simulink library "HEV_Battery_Lib"  (R2024b)
settings: Solver=ode45  StartTime=0.0  StopTime=10.0  RelTol=1e-3  EnableMultiTasking=on
undefined symbols (not defined in the file or in its folder): HEV_Param, Hydride, Kt_Temps, Metal, Nickel
libraries: fl_lib x58, nesl_utility x35, LeadAcidBattery_lib x8, $bdroot x5, Rcecm_lib x4, batteryecm_lib x3, Capacitors_lib x1, spsBatteryLib x1, simulink_extras x1, spsGroundLib x1, spsControlledCurrentSourceLib x1, spsVoltageMeasurementLib x1
(part 2 of 2)

== system HEV_Battery_Lib/Cells/Battery cell2/Thermal Model ==
  Battery thermal mass : fl_lib/Thermal/Thermal Elements/Thermal Mass  mass_type=foundation.enum.constant_variable.constant  mass=1 kg  sp_heat=HEV_Param.Battery_Cell.Ctheta J/kg/K  mass_min=1e-6 kg  num_ports=foundation.enum.numPorts2.one  m_specify=off  m_priority=High  m=1 kg  m_nominal_specify=off  m_nominal_value=1  m_nominal_unit=kg  T_specify=on  T_priority=High  T=HEV_Param.Battery_Cell.theta_init+273 K  T_nominal_specify=off  T_nominal_value=1  T_nominal_unit=K  Q_specify=off  Q_priority=High  Q=0 J/s  Q_nominal_specify=off  Q_nominal_value=1  Q_nominal_unit=J/s
  Ideal Temperature Sensor : fl_lib/Thermal/Thermal Sensors/Temperature Sensor  temperature_measure=foundation.enum.MeasurementReference.difference
  Ideal Heat Flow Source : fl_lib/Thermal/Thermal Sources/Controlled Heat Flow Rate Source
  Kt as a function of temperature : fl_lib/Physical Signals/Lookup Tables/PS Lookup Table (1D)  x=[HEV_Param.Battery_Cell.theta_f,HEV_Param.Battery_Cell. Kt_Temps]+273 K  f=[0 HEV_Param.Battery_Cell.Kt]  interp_method=simscape.enum.interpolation.linear  extrap_method=simscape.enum.extrapolation.linear
  Thermal Reference1 : fl_lib/Thermal/Thermal Elements/Thermal Reference
  Thermal Reference2 : fl_lib/Thermal/Thermal Elements/Thermal Reference
  Ps : PMIOPort  Tag=PMCPort  Side=Left
  H : PMIOPort  Tag=PMCPort  Port=2  Side=Left
  Kt : PMIOPort  Tag=PMCPort  Port=3  Side=Right
  T : PMIOPort  Tag=PMCPort  Port=4  Side=Right
  connections:
  Ideal Heat Flow Source/RConn1 -- Ps/RConn1
  Kt/RConn1 -- Kt as a function of temperature/RConn1
  Battery thermal mass/LConn1 -- Ideal Heat Flow Source/LConn1 -- Ideal Temperature Sensor/LConn1 -- H/RConn1
  Thermal Reference1/LConn1 -- Ideal Heat Flow Source/RConn2
  T/RConn1 -- Kt as a function of temperature/LConn1 -- Ideal Temperature Sensor/RConn2
  Ideal Temperature Sensor/RConn1 -- Thermal Reference2/LConn1

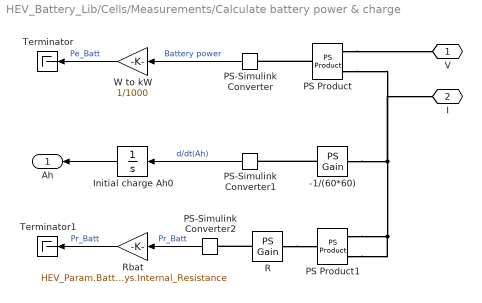
== system HEV_Battery_Lib/Cells/Measurements/Calculate battery power & charge ==
  -1/(60*60) : fl_lib/Physical Signals/Functions/PS Gain  gain=-1/(60*60)
  Initial charge Ah0 : Integrator  InitialCondition=HEV_Param.Battery_Sys.Maximum_Capacity
  PS Product : fl_lib/Physical Signals/Functions/PS Product
  PS Product1 : fl_lib/Physical Signals/Functions/PS Product
  PS-Simulink Converter : nesl_utility/PS-Simulink Converter  PhysicalDomain=network_engine_domain  SubClassName=ps_output  LeftPortType=input  RightPortType=output  PseudoPeriodic=off  Frequencies=[]  VectorFormat=1-D array  Unit=W  AffineConversion=off
  PS-Simulink Converter1 : nesl_utility/PS-Simulink Converter  PhysicalDomain=network_engine_domain  SubClassName=ps_output  LeftPortType=input  RightPortType=output  PseudoPeriodic=off  Frequencies=[]  VectorFormat=1-D array  Unit=A  AffineConversion=off
  PS-Simulink Converter2 : nesl_utility/PS-Simulink Converter  PhysicalDomain=network_engine_domain  SubClassName=ps_output  LeftPortType=input  RightPortType=output  PseudoPeriodic=off  Frequencies=[]  VectorFormat=1-D array  Unit=W  AffineConversion=off
  R : fl_lib/Physical Signals/Functions/PS Gain  gain=HEV_Param.Battery_Sys.Internal_Resistance Ohm
  Rbat : Gain  Gain=HEV_Param.Battery_Sys.Internal_Resistance
  Terminator : Terminator
  Terminator1 : Terminator
  W to kW : Gain  Gain=1/1000
  V : PMIOPort  Side=Left
  I : PMIOPort  Port=2  Side=Left
  Ah : Outport  VectorParamsAs1DForOutWhenUnconnected=off
  wires:
  Rbat/1 -> Terminator1/1  "Pr_Batt"
  Initial charge Ah0/1 -> Ah/1
  W to kW/1 -> Terminator/1  "Pe_Batt"
  PS-Simulink Converter1/1 -> Initial charge Ah0/1  "d/dt(Ah)"
  PS-Simulink Converter2/1 -> Rbat/1  "Pr_Batt"
  PS-Simulink Converter/1 -> W to kW/1  "Battery power"
  connections:
  -1/(60*60)/LConn1 -- PS Product/LConn2 -- I/RConn1 -- PS Product1/LConn2 -- PS Product1/LConn1
  PS Product/LConn1 -- V/RConn1
  R/LConn1 -- PS Product1/RConn1
  -1/(60*60)/RConn1 -- PS-Simulink Converter1/LConn1
  R/RConn1 -- PS-Simulink Converter2/LConn1
  PS Product/RConn1 -- PS-Simulink Converter/LConn1

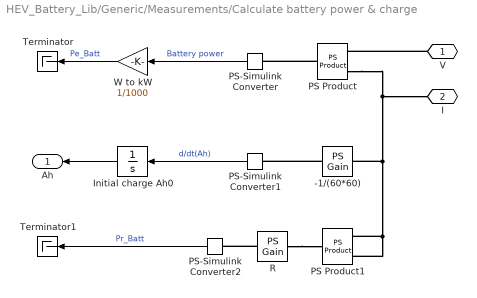
== system HEV_Battery_Lib/Generic/Measurements/Calculate battery power & charge ==
  -1/(60*60) : fl_lib/Physical Signals/Functions/PS Gain  gain=-1/(60*60)
  Initial charge Ah0 : Integrator  InitialCondition=HEV_Param.Battery_Sys.Maximum_Capacity
  PS Product : fl_lib/Physical Signals/Functions/PS Product
  PS Product1 : fl_lib/Physical Signals/Functions/PS Product
  PS-Simulink Converter : nesl_utility/PS-Simulink Converter  PhysicalDomain=network_engine_domain  SubClassName=ps_output  LeftPortType=input  RightPortType=output  PseudoPeriodic=off  Frequencies=[]  VectorFormat=1-D array  Unit=W  AffineConversion=off
  PS-Simulink Converter1 : nesl_utility/PS-Simulink Converter  PhysicalDomain=network_engine_domain  SubClassName=ps_output  LeftPortType=input  RightPortType=output  PseudoPeriodic=off  Frequencies=[]  VectorFormat=1-D array  Unit=A  AffineConversion=off
  PS-Simulink Converter2 : nesl_utility/PS-Simulink Converter  PhysicalDomain=network_engine_domain  SubClassName=ps_output  LeftPortType=input  RightPortType=output  PseudoPeriodic=off  Frequencies=[]  VectorFormat=1-D array  Unit=W  AffineConversion=off
  R : fl_lib/Physical Signals/Functions/PS Gain  gain=HEV_Param.Battery_Sys.Internal_Resistance Ohm
  Terminator : Terminator
  Terminator1 : Terminator
  W to kW : Gain  Gain=1/1000
  V : PMIOPort  Side=Left
  I : PMIOPort  Port=2  Side=Left
  Ah : Outport  VectorParamsAs1DForOutWhenUnconnected=off
  wires:
  PS-Simulink Converter/1 -> W to kW/1  "Battery power"
  W to kW/1 -> Terminator/1  "Pe_Batt"
  PS-Simulink Converter1/1 -> Initial charge Ah0/1  "d/dt(Ah)"
  Initial charge Ah0/1 -> Ah/1
  PS-Simulink Converter2/1 -> Terminator1/1  "Pr_Batt"
  connections:
  R/RConn1 -- PS-Simulink Converter2/LConn1
  PS Product/RConn1 -- PS-Simulink Converter/LConn1
  V/RConn1 -- PS Product/LConn1
  PS Product/LConn2 -- I/RConn1 -- -1/(60*60)/LConn1 -- PS Product1/LConn1 -- PS Product1/LConn2
  -1/(60*60)/RConn1 -- PS-Simulink Converter1/LConn1
  R/LConn1 -- PS Product1/RConn1

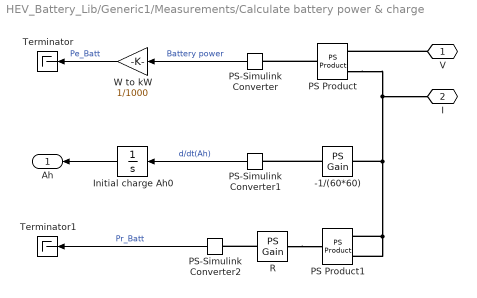
== system HEV_Battery_Lib/Generic1/Measurements/Calculate battery power & charge ==
  -1/(60*60) : fl_lib/Physical Signals/Functions/PS Gain  gain=-1/(60*60)
  Initial charge Ah0 : Integrator  InitialCondition=HEV_Param.Battery_Sys.Maximum_Capacity
  PS Product : fl_lib/Physical Signals/Functions/PS Product
  PS Product1 : fl_lib/Physical Signals/Functions/PS Product
  PS-Simulink Converter : nesl_utility/PS-Simulink Converter  PhysicalDomain=network_engine_domain  SubClassName=ps_output  LeftPortType=input  RightPortType=output  PseudoPeriodic=off  Frequencies=[]  VectorFormat=1-D array  Unit=W  AffineConversion=off
  PS-Simulink Converter1 : nesl_utility/PS-Simulink Converter  PhysicalDomain=network_engine_domain  SubClassName=ps_output  LeftPortType=input  RightPortType=output  PseudoPeriodic=off  Frequencies=[]  VectorFormat=1-D array  Unit=A  AffineConversion=off
  PS-Simulink Converter2 : nesl_utility/PS-Simulink Converter  PhysicalDomain=network_engine_domain  SubClassName=ps_output  LeftPortType=input  RightPortType=output  PseudoPeriodic=off  Frequencies=[]  VectorFormat=1-D array  Unit=W  AffineConversion=off
  R : fl_lib/Physical Signals/Functions/PS Gain  gain=HEV_Param.Battery_Sys.Internal_Resistance Ohm
  Terminator : Terminator
  Terminator1 : Terminator
  W to kW : Gain  Gain=1/1000
  V : PMIOPort  Side=Left
  I : PMIOPort  Port=2  Side=Left
  Ah : Outport  VectorParamsAs1DForOutWhenUnconnected=off
  wires:
  PS-Simulink Converter/1 -> W to kW/1  "Battery power"
  W to kW/1 -> Terminator/1  "Pe_Batt"
  PS-Simulink Converter1/1 -> Initial charge Ah0/1  "d/dt(Ah)"
  Initial charge Ah0/1 -> Ah/1
  PS-Simulink Converter2/1 -> Terminator1/1  "Pr_Batt"
  connections:
  R/RConn1 -- PS-Simulink Converter2/LConn1
  PS Product/RConn1 -- PS-Simulink Converter/LConn1
  V/RConn1 -- PS Product/LConn1
  PS Product/LConn2 -- I/RConn1 -- -1/(60*60)/LConn1 -- PS Product1/LConn1 -- PS Product1/LConn2
  -1/(60*60)/RConn1 -- PS-Simulink Converter1/LConn1
  R/LConn1 -- PS Product1/RConn1

== system HEV_Battery_Lib/Predefined/GF1/SOC Offset ==
  note: For control logic to work consistently
      | for all versions, SOC% must be scaled
  In1 : Inport
  Bus Creator : BusCreator  Inputs=4
  Bus Selector : BusSelector  OutputSignals=SOC (%)
  Bus Selector1 : BusSelector  OutputSignals=Current (A),Voltage (V)
  Gain : Gain  Gain=100/HEV_Param.Battery_Det.Initial_SOC
  Gain1 : Gain  Gain=-1/(60*60)
  Initial charge Ah0 : Integrator  InitialCondition=HEV_Param.Battery_Det.Rated_Capacity*HEV_Param.Battery_Det.Initial_SOC/100
  Transfer Fcn (with initial states) : simulink_extras/Additional Linear/Transfer Fcn (with initial states)  N=[1]  D="[0.01  1]"  X0=100/HEV_Param.Battery_Det.Initial_SOC
  Out1 : Outport  VectorParamsAs1DForOutWhenUnconnected=off
  wires:
  In1/1 -> Bus Selector/1, Bus Selector1/1
  Bus Selector/1 -> Gain/1  "<SOC (%)>"
  Bus Selector1/1 -> Bus Creator/2, Gain1/1  "<Current (A)>"
  Gain/1 -> Transfer Fcn (with initial states)/1  "SOC (%)"
  Bus Selector1/2 -> Bus Creator/3  "<Voltage (V)>"
  Bus Creator/1 -> Out1/1
  Gain1/1 -> Initial charge Ah0/1
  Initial charge Ah0/1 -> Bus Creator/1  "Batt_Ah"
  Transfer Fcn (with initial states)/1 -> Bus Creator/4  "SOC (%)"

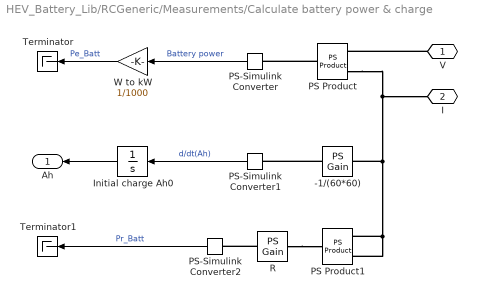
== system HEV_Battery_Lib/RCGeneric/Measurements/Calculate battery power & charge ==
  -1/(60*60) : fl_lib/Physical Signals/Functions/PS Gain  gain=-1/(60*60)
  Initial charge Ah0 : Integrator  InitialCondition=HEV_Param.Battery_Sys.Maximum_Capacity
  PS Product : fl_lib/Physical Signals/Functions/PS Product
  PS Product1 : fl_lib/Physical Signals/Functions/PS Product
  PS-Simulink Converter : nesl_utility/PS-Simulink Converter  PhysicalDomain=network_engine_domain  SubClassName=ps_output  LeftPortType=input  RightPortType=output  PseudoPeriodic=off  Frequencies=[]  VectorFormat=1-D array  Unit=W  AffineConversion=off
  PS-Simulink Converter1 : nesl_utility/PS-Simulink Converter  PhysicalDomain=network_engine_domain  SubClassName=ps_output  LeftPortType=input  RightPortType=output  PseudoPeriodic=off  Frequencies=[]  VectorFormat=1-D array  Unit=A  AffineConversion=off
  PS-Simulink Converter2 : nesl_utility/PS-Simulink Converter  PhysicalDomain=network_engine_domain  SubClassName=ps_output  LeftPortType=input  RightPortType=output  PseudoPeriodic=off  Frequencies=[]  VectorFormat=1-D array  Unit=W  AffineConversion=off
  R : fl_lib/Physical Signals/Functions/PS Gain  gain=HEV_Param.Battery_Sys.Internal_Resistance Ohm
  Terminator : Terminator
  Terminator1 : Terminator
  W to kW : Gain  Gain=1/1000
  V : PMIOPort  Side=Left
  I : PMIOPort  Port=2  Side=Left
  Ah : Outport  VectorParamsAs1DForOutWhenUnconnected=off
  wires:
  PS-Simulink Converter/1 -> W to kW/1  "Battery power"
  W to kW/1 -> Terminator/1  "Pe_Batt"
  PS-Simulink Converter1/1 -> Initial charge Ah0/1  "d/dt(Ah)"
  Initial charge Ah0/1 -> Ah/1
  PS-Simulink Converter2/1 -> Terminator1/1  "Pr_Batt"
  connections:
  R/RConn1 -- PS-Simulink Converter2/LConn1
  PS Product/RConn1 -- PS-Simulink Converter/LConn1
  V/RConn1 -- PS Product/LConn1
  PS Product/LConn2 -- I/RConn1 -- -1/(60*60)/LConn1 -- PS Product1/LConn1 -- PS Product1/LConn2
  -1/(60*60)/RConn1 -- PS-Simulink Converter1/LConn1
  R/LConn1 -- PS Product1/RConn1
